simulink model "linearmod"  (R2024b)
settings: Solver=FixedStepAuto  StartTime=0.0  StopTime=T  RelTol=1e-3
values from neighbouring files (symbols this model uses):
  A = sys_d.A    [CrazyP2P.m]    (also in Drone4into12.m; ILCLinear.m; Tuning_script.m; p2p.m)
  B = sys_d.B    [CrazyP2P.m]    (also in Drone4into12.m; ILCLinear.m; Tuning_script.m; p2p.m)
  C = sys_d.C    [CrazyP2P.m]    (also in Drone4into12.m; ILCLinear.m; Tuning_script.m; p2p.m)
  D = sys_d.D    [CrazyP2P.m]    (also in Drone4into12.m; ILCLinear.m; Tuning_script.m; p2p.m)
  Ts = 1/100    (= 0.01)    [CrazyP2P.m]    (also in Drone4into12.m; ILCLinear.m; Tuning_script.m; p2p.m)
settings Model: Creator=ellio  LastModifiedBy=ellio

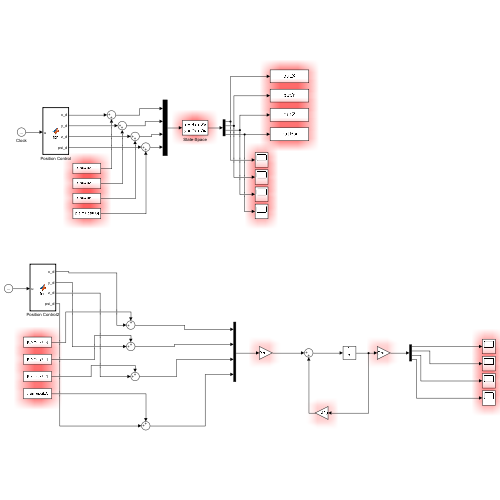
[thumbnail: Simulink's stored preview of the top-level diagram]
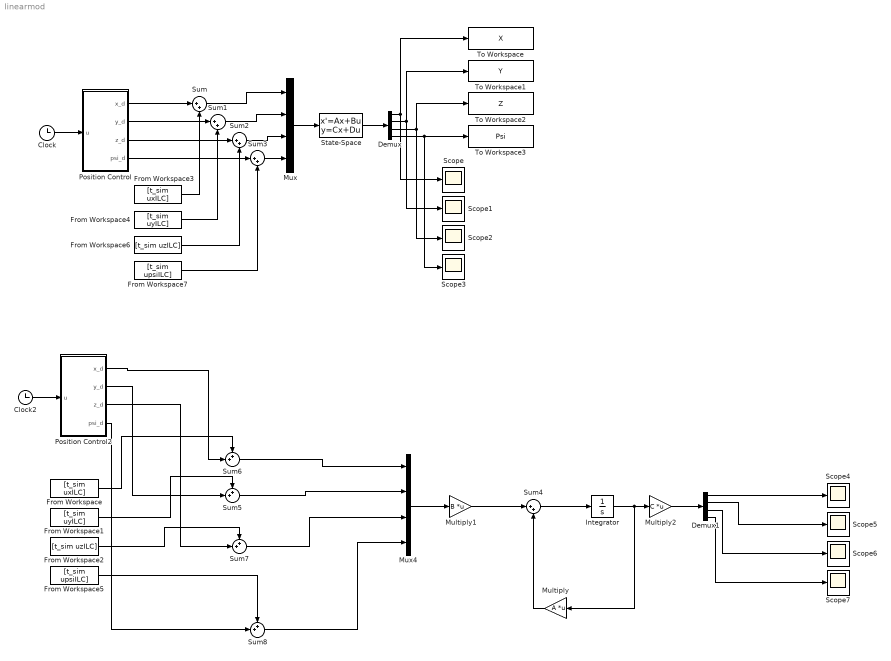
== system linearmod ==
  Clock : Clock
  Clock2 : Clock
  Demux : Demux
  Demux1 : Demux
  From Workspace : FromWorkspace  VariableName=[t_sim uxILC]  SampleTime=Ts
  From Workspace1 : FromWorkspace  VariableName=[t_sim uyILC]  SampleTime=Ts
  From Workspace2 : FromWorkspace  VariableName=[t_sim uzILC]  SampleTime=Ts
  From Workspace3 : FromWorkspace  VariableName=[t_sim uxILC]  SampleTime=Ts
  From Workspace4 : FromWorkspace  VariableName=[t_sim uyILC]  SampleTime=Ts
  From Workspace5 : FromWorkspace  VariableName=[t_sim upsiILC]  SampleTime=Ts
  From Workspace6 : FromWorkspace  VariableName=[t_sim uzILC]  SampleTime=Ts
  From Workspace7 : FromWorkspace  VariableName=[t_sim upsiILC]  SampleTime=Ts
  Integrator : Integrator
  Multiply : Gain  Gain=A  Multiplication=Matrix(K*u)
  Multiply1 : Gain  Gain=B  Multiplication=Matrix(K*u)
  Multiply2 : Gain  Gain=C  Multiplication=Matrix(K*u)
  Mux : Mux
  Mux4 : Mux
  Position Control : MATLAB Function  TreatAsAtomicUnit=on
  Position Control2 : MATLAB Function  TreatAsAtomicUnit=on
  Scope{,1..7} (8 alike) : Scope
  State-Space : StateSpace  A=A  B=B  C=C  D=D  InitialCondition=0
  Sum{,1..4} (5 alike) : Sum  Inputs=|++
  Sum{5..8} (4 alike) : Sum  Inputs=++|
  To Workspace : ToWorkspace  VariableName=X  SampleTime=Ts
  To Workspace1 : ToWorkspace  VariableName=Y  SampleTime=Ts
  To Workspace2 : ToWorkspace  VariableName=Z  SampleTime=Ts
  To Workspace3 : ToWorkspace  VariableName=Psi  SampleTime=Ts
  wires:
  Mux/1 -> State-Space/1
  State-Space/1 -> Demux/1
  Demux/1 -> To Workspace/1, Scope/1
  Demux/2 -> To Workspace1/1, Scope1/1
  Demux/3 -> To Workspace2/1, Scope2/1
  Demux/4 -> Scope3/1, To Workspace3/1
  Position Control/1(x_d) -> Sum/1
  Sum/1 -> Mux/1
  From Workspace/1 -> Sum6/1
  Position Control/2(y_d) -> Sum1/1
  Sum1/1 -> Mux/2
  From Workspace1/1 -> Sum5/1
  Position Control/3(z_d) -> Sum2/1
  Sum2/1 -> Mux/3
  From Workspace2/1 -> Sum7/1
  Position Control/4(psi_d) -> Sum3/1
  Sum3/1 -> Mux/4
  From Workspace5/1 -> Sum8/1
  Multiply1/1 -> Sum4/1
  Multiply/1 -> Sum4/2
  Sum4/1 -> Integrator/1
  Integrator/1 -> Multiply2/1, Multiply/1
  Position Control2/4(psi_d) -> Sum8/2
  Position Control2/3(z_d) -> Sum7/2
  Clock2/1 -> Position Control2/1(u)
  Position Control2/2(y_d) -> Sum5/2
  Position Control2/1(x_d) -> Sum6/2
  Sum6/1 -> Mux4/1
  Sum5/1 -> Mux4/2
  Sum7/1 -> Mux4/3
  Sum8/1 -> Mux4/4
  Demux1/3 -> Scope6/1
  Multiply2/1 -> Demux1/1
  Demux1/1 -> Scope4/1
  Demux1/2 -> Scope5/1
  Demux1/4 -> Scope7/1
  Mux4/1 -> Multiply1/1
  From Workspace4/1 -> Sum1/2
  From Workspace3/1 -> Sum/2
  From Workspace6/1 -> Sum2/2
  From Workspace7/1 -> Sum3/2
  Clock/1 -> Position Control/1(u)

== matlab function linearmod/Position Control ==
  data: u input; x_d output; y_d output; z_d output; psi_d output
function [x_d,y_d,z_d,psi_d] = fcn(u)
    %mine
    x_d = 1 - cos(2 * u);
    y_d = sin(2 * u);
    z_d = 2 * u;
    psi_d = 0*u;

%%%%%%%%%%%% OG %%%%%%%%%%%
    %x_d = 0.5*(1-cos(2*u));%1;
    %y_d = 0.5*sin(2*u);%1;
    %z_d = 0.1*u;%-5*9.81*u^2;
    %psi_d = 0;
end

== matlab function linearmod/Position Control2 ==
  data: u input; x_d output; y_d output; z_d output; psi_d output
function [x_d,y_d,z_d,psi_d] = fcn(u)
    %mine
    x_d = 1 - cos(2 * u);
    y_d = sin(2 * u);
    z_d = 2 * u;
    psi_d = 0*u;

%%%%%%%%%%%% OG %%%%%%%%%%%
    %x_d = 0.5*(1-cos(2*u));%1;
    %y_d = 0.5*sin(2*u);%1;
    %z_d = 0.1*u;%-5*9.81*u^2;
    %psi_d = 0;
end
